simulink library "hal"  (Simulink 8.2)
settings: Solver=ode45  SolverMode=SingleTasking  StartTime=0.0  StopTime=10.0  RelTol=1e-3
PostLoadFcn:
  | , if any(exist('dsrtsu_mdlpostloadfcn', 'file') == [2, 3, 6]), try dsrtsu_mdlpostloadfcn('Execute', bdroot); catch fprintf('Error in PostLoadFcn (dsrtsu_mdlpostloadfcn) for model "%s":\n %s\n', bdroot, lasterr); end, end,
values from neighbouring files (symbols this model uses):
  INVALID_ABS1_TIMEOUT = single(0.03)    [hal_def.m]
  INVALID_ABS2_TIMEOUT = single(0.03)    [hal_def.m]
  INVALID_ABS3_TIMEOUT = single(0.03)    [hal_def.m]
  INVALID_ABS4_TIMEOUT = single(0.03)    [hal_def.m]
  INVALID_AC1_TIMEOUT = single(0.3)    [hal_def.m]
  INVALID_BCM1_TIMEOUT = single(0.6)    [hal_def.m]
  INVALID_BCM2_TIMEOUT = single(0.06)    [hal_def.m]
  INVALID_BOOSTER_VAC = uint32(255)    [hal_def.m]
  INVALID_CUR_VEHDECE = uint32(255)    [hal_def.m]
  INVALID_CURBRAKEDECE_REQ = uint32(255)    [hal_def.m]
  INVALID_CURSTEERANG_REQ = uint32(65535)    [hal_def.m]
  INVALID_CURSTEERTQ_REQ = uint32(255)    [hal_def.m]
  INVALID_ECM1_TIMEOUT = single(0.03)    [hal_def.m]
  INVALID_ECM2_TIMEOUT = single(0.03)    [hal_def.m]
  INVALID_ECM3_TIMEOUT = single(0.03)    [hal_def.m]
  INVALID_ECM9_TIMEOUT = single(0.03)    [hal_def.m]
  INVALID_ENG_TORQUE_FRICTIONAL = uint32(255)    [hal_def.m]
  INVALID_ENG_TORQUE_INDICATED = uint32(255)    [hal_def.m]
  INVALID_ENG_TORQUE_INDICATEDCOR = uint32(255)    [hal_def.m]
  INVALID_ENG_TQ_MAX = uint32(65535)    [hal_def.m]
  INVALID_ENG_TQ_MIN = uint32(65535)    [hal_def.m]
  INVALID_EPAS2_TIMEOUT = single(0.03)    [hal_def.m]
  INVALID_EPAS3_TIMEOUT = single(0.03)    [hal_def.m]
  INVALID_EPB1_TIMEOUT = single(0.12)    [hal_def.m]
  INVALID_EPS_BATTVOLT = uint32(251)    [hal_def.m]
  INVALID_ESC_BATTVOLT = uint32(251)    [hal_def.m]
  INVALID_GRADE = uint32(255)    [hal_def.m]
  INVALID_HCU3_TIMEOUT = single(0.03)    [hal_def.m]
  INVALID_HCU4_TIMEOUT = single(0.03)    [hal_def.m]
  INVALID_HMI1_TIMEOUT = single(0.03)    [hal_def.m]
  INVALID_HMI2_TIMEOUT = single(0.03)    [hal_def.m]
  INVALID_LAT_ACC = uint32(255)    [hal_def.m]
  INVALID_LONG_ACC = uint32(255)    [hal_def.m]
  INVALID_MC_PRESSURE = uint32(2047)    [hal_def.m]
  INVALID_METER1_TIMEOUT = single(0.3)    [hal_def.m]
  INVALID_METER3_TIMEOUT = single(0.3)    [hal_def.m]
  INVALID_METER_VEHSPD = uint32(2048)    [hal_def.m]
  INVALID_ODO_METER = uint32(1000000)    [hal_def.m]
  INVALID_OUTSIDE_TEMP = uint32(96)    [hal_def.m]
  INVALID_PARKBRAKEBIND_STAT = uint32(3)    [hal_def.m]
  INVALID_SAS1_TIMEOUT = single(0.03)    [hal_def.m]
  INVALID_SAS_ANGLE = uint32(65535)    [hal_def.m]
  INVALID_SHIFTER_POSN = uint32(6)    [hal_def.m]
  INVALID_TCM1_TIMEOUT = single(0.03)    [hal_def.m]
  INVALID_TCM2_TIMEOUT = single(0.03)    [hal_def.m]
  INVALID_VCU1_TIMEOUT = single(0.03)    [hal_def.m]
  INVALID_VCU2_TIMEOUT = single(0.03)    [hal_def.m]
  INVALID_VEH_CRASH = uint32(15)    [hal_def.m]
  INVALID_VEH_SPD = uint32(2048)    [hal_def.m]
  INVALID_WHEEL_SPD = uint32(16377)    [hal_def.m]
  INVALID_YAW_RATE = uint32(2001)    [hal_def.m]
undefined symbols (not defined in the file or in its folder): C_TASK_5MS_S, FALSE, INVALID_CURPTTORQ_REQ, KHAL_MssgIdObj1_num, KHAL_MssgIdObj2_num, KHAL_MssgIdObjStatus_num, TRUE
libraries: simulink x92
(part 6 of 8)

== system hal/dHAL_IN/dHAL_IN_ECM ==
  CAN1_Rx : Inport
  BO_790_ECM1_8_ECM : Subsystem
  BO_809_ECM2_8_ECM : Subsystem
  BO_821_ECM3_8_ECM : Subsystem
  BO_875_ECM9_8_ECM : Subsystem
  KFUN_AStpTimeMin_s1 : Constant  Value=INVALID_ENG_TORQUE_INDICATED
  KFUN_AStpTimeMin_s2 : Constant  Value=INVALID_ENG_TORQUE_INDICATEDCOR
  KFUN_AStpTimeMin_s3 : Constant  Value=INVALID_ENG_TORQUE_FRICTIONAL
  KFUN_AStpTimeMin_s5 : Constant  Value=INVALID_ENG_TQ_MAX
  KFUN_AStpTimeMin_s6 : Constant  Value=INVALID_ENG_TQ_MIN
  Relational Operator{1..3,5..6} (5 alike) : RelationalOperator  OutDataTypeStr=boolean
  VHAL_AccelPedalPosn_pct : Outport
  VHAL_AccelPedalPosnInvalid_flg : Outport  Port=2
  VHAL_EffAccelPedalPosn_pct : Outport  Port=3
  VHAL_EffAccelPedalPosnInvalid_flg : Outport  Port=4
  VHAL_CCEnable_flg : Outport  Port=5
  VHAL_CCEnableInvalid_flg : Outport  Port=6
  VHAL_CCActive_flg : Outport  Port=7
  VHAL_CCActiveInvalid_flg : Outport  Port=8
  VHAL_EngSpd_erpm : Outport  Port=9
  VHAL_EngSpdInvalid_flg : Outport  Port=10
  VHAL_EngTqIndicated_Nm : Outport  Port=11
  VHAL_EngTqIndicatedInvalid_flg : Outport  Port=12
  VHAL_EngTqIndicatedCOR_Nm : Outport  Port=13
  VHAL_EngTqIndicatedCORInvalid_flg : Outport  Port=14
  VHAL_EngTqUnCORFault_flg : Outport  Port=15
  VHAL_EngTqFriction_Nm : Outport  Port=16
  VHAL_EngTqFrictionInvalid_flg : Outport  Port=17
  VHAL_StandardTq_Nm : Outport  Port=18
  VHAL_EngTqMax_Nm : Outport  Port=19
  VHAL_EngTqMaxInvalid_flg : Outport  Port=20
  VHAL_EngTqMin_Nm : Outport  Port=21
  VHAL_EngTqMinInvalid_flg : Outport  Port=22
  VHAL_EMSHybridOpState_enum : Outport  Port=23
  VHAL_EMSOpState_enum : Outport  Port=24
  VHAL_ECM9RollCnt_cnt : Outport  Port=25
  VHAL_EngHoodOpen_flg : Outport  Port=26
  VHAL_EngRunning_flg : Outport  Port=27
  wires:
  BO_875_ECM9_8_ECM/7(EngTqMin_raw) -> Relational Operator6/1
  BO_875_ECM9_8_ECM/6(EngTqMin) -> VHAL_EngTqMin_Nm/1
  BO_875_ECM9_8_ECM/5(EngTqMax_raw) -> Relational Operator5/1
  BO_790_ECM1_8_ECM/7(CAN_TQI_ACOR_raw) -> Relational Operator2/1
  BO_790_ECM1_8_ECM/5(CAN_TQI_raw) -> Relational Operator1/1
  BO_790_ECM1_8_ECM/3(CAN_TQFR_raw) -> Relational Operator3/1
  KFUN_AStpTimeMin_s5/1 -> Relational Operator5/2
  KFUN_AStpTimeMin_s6/1 -> Relational Operator6/2
  KFUN_AStpTimeMin_s3/1 -> Relational Operator3/2
  KFUN_AStpTimeMin_s1/1 -> Relational Operator1/2
  KFUN_AStpTimeMin_s2/1 -> Relational Operator2/2
  BO_809_ECM2_8_ECM/1(Eng_Hood_SW) -> VHAL_EngHoodOpen_flg/1
  BO_809_ECM2_8_ECM/2(LV_CAN_ENG_RUN_ST) -> VHAL_EngRunning_flg/1
  [CAN1_Rx] -> BO_809_ECM2_8_ECM/1(CAN1_Rx)
  BO_875_ECM9_8_ECM/1(ECM9RollCnt) -> VHAL_ECM9RollCnt_cnt/1
  BO_875_ECM9_8_ECM/2(EMSHybridOpState) -> VHAL_EMSHybridOpState_enum/1
  BO_875_ECM9_8_ECM/3(EMSOpState) -> VHAL_EMSOpState_enum/1
  BO_875_ECM9_8_ECM/4(EngTqMax) -> VHAL_EngTqMax_Nm/1
  Relational Operator5/1 -> VHAL_EngTqMaxInvalid_flg/1
  Relational Operator6/1 -> VHAL_EngTqMinInvalid_flg/1
  [CAN1_Rx] -> BO_875_ECM9_8_ECM/1(CAN1_Rx1)
  Relational Operator3/1 -> VHAL_EngTqFrictionInvalid_flg/1
  BO_790_ECM1_8_ECM/2(CAN_TQFR) -> VHAL_EngTqFriction_Nm/1
  BO_790_ECM1_8_ECM/8(CAN_TQ_STND) -> VHAL_StandardTq_Nm/1
  BO_790_ECM1_8_ECM/9(LV_CAN_N_ERR) -> VHAL_EngSpdInvalid_flg/1
  BO_790_ECM1_8_ECM/1(CAN_N) -> VHAL_EngSpd_erpm/1
  Relational Operator1/1 -> VHAL_EngTqIndicatedInvalid_flg/1
  BO_790_ECM1_8_ECM/4(CAN_TQI) -> VHAL_EngTqIndicated_Nm/1
  BO_790_ECM1_8_ECM/6(CAN_TQI_ACOR) -> VHAL_EngTqIndicatedCOR_Nm/1
  Relational Operator2/1 -> VHAL_EngTqIndicatedCORInvalid_flg/1
  BO_790_ECM1_8_ECM/10(LV_CAN_SUB_TQI) -> VHAL_EngTqUnCORFault_flg/1
  [CAN1_Rx] -> BO_790_ECM1_8_ECM/1(CAN1_Rx)
  BO_821_ECM3_8_ECM/1(CAN_PV_AV) -> VHAL_AccelPedalPosn_pct/1
  BO_821_ECM3_8_ECM/2(CAN_PV_EFC) -> VHAL_EffAccelPedalPosn_pct/1
  BO_821_ECM3_8_ECM/3(LV_CAN_ERRPAS) -> VHAL_AccelPedalPosnInvalid_flg/1
  BO_821_ECM3_8_ECM/4(LV_CAN_ERRPVS) -> VHAL_EffAccelPedalPosnInvalid_flg/1
  BO_821_ECM3_8_ECM/5(LV_CAN_MAIN_CRU) -> VHAL_CCEnable_flg/1
  BO_821_ECM3_8_ECM/6(LV_CAN_MAIN_CRU_ER) -> VHAL_CCEnableInvalid_flg/1
  BO_821_ECM3_8_ECM/7(LV_CAN_SET_CRU) -> VHAL_CCActive_flg/1
  BO_821_ECM3_8_ECM/8(LV_CAN_SET_CRU_ERR) -> VHAL_CCActiveInvalid_flg/1
  [CAN1_Rx] -> BO_821_ECM3_8_ECM/1(CAN1_Rx)
  CAN1_Rx/1 -> [CAN1_Rx]

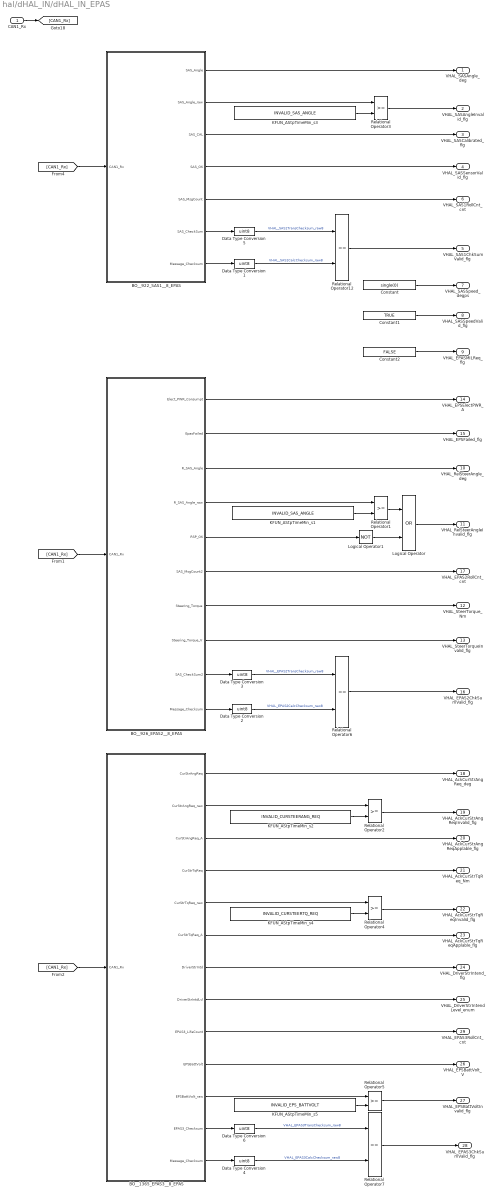
== system hal/dHAL_IN/dHAL_IN_EPAS ==
  CAN1_Rx : Inport
  BO__1365_EPAS3__8_EPAS : Subsystem
  BO__922_SAS1__8_EPAS : Subsystem
  BO__926_EPAS2__8_EPAS : Subsystem
  Constant : Constant  Value=single(0)
  Constant1 : Constant  Value=TRUE
  Constant2 : Constant  Value=FALSE
  Data Type Conversion{1..6} (6 alike) : DataTypeConversion  OutDataTypeStr=uint8
  KFUN_AStpTimeMin_s1 : Constant  Value=INVALID_SAS_ANGLE
  KFUN_AStpTimeMin_s2 : Constant  Value=INVALID_CURSTEERANG_REQ
  KFUN_AStpTimeMin_s3 : Constant  Value=INVALID_SAS_ANGLE
  KFUN_AStpTimeMin_s4 : Constant  Value=INVALID_CURSTEERTQ_REQ
  KFUN_AStpTimeMin_s5 : Constant  Value=INVALID_EPS_BATTVOLT
  Logical Operator : Logic  Operator=OR  AllPortsSameDT=off  OutDataTypeStr=boolean
  Logical Operator1 : Logic  Operator=NOT  AllPortsSameDT=off  OutDataTypeStr=boolean
  Relational Operator{1..5} (5 alike) : RelationalOperator  OutDataTypeStr=boolean
  Relational Operator12 : RelationalOperator  Operator===  OutDataTypeStr=boolean
  Relational Operator6 : RelationalOperator  Operator===  OutDataTypeStr=boolean
  Relational Operator7 : RelationalOperator  Operator===  OutDataTypeStr=boolean
  VHAL_SASAngle_deg : Outport
  VHAL_SASAngleInvalid_flg : Outport  Port=2
  VHAL_SASCalibrated_flg : Outport  Port=3
  VHAL_SASSensorValid_flg : Outport  Port=4
  VHAL_SAS1ChkSumValid_flg : Outport  Port=5
  VHAL_SAS1RollCnt_cnt : Outport  Port=6
  VHAL_SASSpeed_degps : Outport  Port=7
  VHAL_SASSpeedValid_flg : Outport  Port=8
  VHAL_EPASMILReq_flg : Outport  Port=9
  VHAL_RelSteerAngle_deg : Outport  Port=10
  VHAL_RelSteerAngleInvalid_flg : Outport  Port=11
  VHAL_SteerTorque_Nm : Outport  Port=12
  VHAL_SteerTorqueInvalid_flg : Outport  Port=13
  VHAL_EPSElectPWR_A : Outport  Port=14
  VHAL_EPSFailed_flg : Outport  Port=15
  VHAL_EPAS2ChkSumValid_flg : Outport  Port=16
  VHAL_EPAS2RollCnt_cnt : Outport  Port=17
  VHAL_AckCurStrAngReq_deg : Outport  Port=18
  VHAL_AckCurStrAngReqInvalid_flg : Outport  Port=19
  VHAL_AckCurStrAngReqApplable_flg : Outport  Port=20
  VHAL_AckCurStrTqReq_Nm : Outport  Port=21
  VHAL_AckCurStrTqReqInvalid_flg : Outport  Port=22
  VHAL_AckCurStrTqReqApplable_flg : Outport  Port=23
  VHAL_DriverStrIntend_flg : Outport  Port=24
  VHAL_DriverStrIntendLevel_enum : Outport  Port=25
  VHAL_EPSBattVolt_V : Outport  Port=26
  VHAL_EPSBattVoltInvalid_flg : Outport  Port=27
  VHAL_EPAS3ChkSumValid_flg : Outport  Port=28
  VHAL_EPAS3RollCnt_cnt : Outport  Port=29
  wires:
  BO__1365_EPAS3__8_EPAS/5(CurStrTqReq_raw) -> Relational Operator4/1
  BO__1365_EPAS3__8_EPAS/11(EPSBattVolt_raw) -> Relational Operator5/1
  BO__1365_EPAS3__8_EPAS/10(EPSBattVolt) -> VHAL_EPSBattVolt_V/1
  BO__1365_EPAS3__8_EPAS/2(CurStrAngReq_raw) -> Relational Operator2/1
  [CAN1_Rx] -> BO__1365_EPAS3__8_EPAS/1(CAN1_Rx)
  BO__926_EPAS2__8_EPAS/4(R_SAS_Angle_raw) -> Relational Operator1/1
  BO__922_SAS1__8_EPAS/2(SAS_Angle_raw) -> Relational Operator3/1
  [CAN1_Rx] -> BO__926_EPAS2__8_EPAS/1(CAN1_Rx)
  [CAN1_Rx] -> BO__922_SAS1__8_EPAS/1(CAN1_Rx)
  CAN1_Rx/1 -> [CAN1_Rx]
  BO__1365_EPAS3__8_EPAS/3(CurStrAngReq_A) -> VHAL_AckCurStrAngReqApplable_flg/1
  BO__1365_EPAS3__8_EPAS/13(Message_Checksum) -> Data Type Conversion4/1
  BO__1365_EPAS3__8_EPAS/12(EPAS3_Checksum) -> Data Type Conversion6/1
  Relational Operator7/1 -> VHAL_EPAS3ChkSumValid_flg/1
  Data Type Conversion4/1 -> Relational Operator7/2  "VHAL_EPAS3CalcChecksum_raw8"
  Data Type Conversion6/1 -> Relational Operator7/1  "VHAL_EPAS3TransChecksum_raw8"
  BO__926_EPAS2__8_EPAS/10(Message_Checksum) -> Data Type Conversion2/1
  BO__926_EPAS2__8_EPAS/9(SAS_CheckSum2) -> Data Type Conversion3/1
  Relational Operator6/1 -> VHAL_EPAS2ChkSumValid_flg/1
  Data Type Conversion2/1 -> Relational Operator6/2  "VHAL_EPAS2CalcChecksum_raw8"
  Data Type Conversion3/1 -> Relational Operator6/1  "VHAL_EPAS2TransChecksum_raw8"
  Relational Operator12/1 -> VHAL_SAS1ChkSumValid_flg/1
  Data Type Conversion1/1 -> Relational Operator12/2  "VHAL_SAS1CalcChecksum_raw8"
  Data Type Conversion5/1 -> Relational Operator12/1  "VHAL_SAS1TransChecksum_raw8"
  BO__922_SAS1__8_EPAS/7(Message_Checksum) -> Data Type Conversion1/1
  BO__922_SAS1__8_EPAS/6(SAS_CheckSum) -> Data Type Conversion5/1
  Relational Operator5/1 -> VHAL_EPSBattVoltInvalid_flg/1
  KFUN_AStpTimeMin_s5/1 -> Relational Operator5/2
  BO__1365_EPAS3__8_EPAS/8(DriverStrIntdLvl) -> VHAL_DriverStrIntendLevel_enum/1
  BO__1365_EPAS3__8_EPAS/7(DriverStrIntd) -> VHAL_DriverStrIntend_flg/1
  BO__1365_EPAS3__8_EPAS/4(CurStrTqReq) -> VHAL_AckCurStrTqReq_Nm/1
  BO__1365_EPAS3__8_EPAS/6(CurStrTqReq_A) -> VHAL_AckCurStrTqReqApplable_flg/1
  Relational Operator4/1 -> VHAL_AckCurStrTqReqInvalid_flg/1
  KFUN_AStpTimeMin_s4/1 -> Relational Operator4/2
  Relational Operator2/1 -> VHAL_AckCurStrAngReqInvalid_flg/1
  KFUN_AStpTimeMin_s2/1 -> Relational Operator2/2
  BO__1365_EPAS3__8_EPAS/1(CurStrAngReq) -> VHAL_AckCurStrAngReq_deg/1
  Logical Operator1/1 -> Logical Operator/2
  Logical Operator/1 -> VHAL_RelSteerAngleInvalid_flg/1
  Relational Operator1/1 -> Logical Operator/1
  KFUN_AStpTimeMin_s1/1 -> Relational Operator1/2
  BO__926_EPAS2__8_EPAS/3(R_SAS_Angle) -> VHAL_RelSteerAngle_deg/1
  Relational Operator3/1 -> VHAL_SASAngleInvalid_flg/1
  BO__922_SAS1__8_EPAS/1(SAS_Angle) -> VHAL_SASAngle_deg/1
  KFUN_AStpTimeMin_s3/1 -> Relational Operator3/2
  BO__926_EPAS2__8_EPAS/8(Steering_Torque_V) -> VHAL_SteerTorqueInvalid_flg/1
  BO__926_EPAS2__8_EPAS/7(Steering_Torque) -> VHAL_SteerTorque_Nm/1
  BO__926_EPAS2__8_EPAS/6(SAS_MsgCount2) -> VHAL_EPAS2RollCnt_cnt/1
  BO__926_EPAS2__8_EPAS/5(RSP_OK) -> Logical Operator1/1
  BO__926_EPAS2__8_EPAS/2(EpasFailed) -> VHAL_EPSFailed_flg/1
  BO__926_EPAS2__8_EPAS/1(Elect_PWR_Consumpt) -> VHAL_EPSElectPWR_A/1
  BO__1365_EPAS3__8_EPAS/9(EPAS3_LifeCount) -> VHAL_EPAS3RollCnt_cnt/1
  BO__922_SAS1__8_EPAS/4(SAS_OK) -> VHAL_SASSensorValid_flg/1
  BO__922_SAS1__8_EPAS/5(SAS_MsgCount) -> VHAL_SAS1RollCnt_cnt/1
  BO__922_SAS1__8_EPAS/3(SAS_CAL) -> VHAL_SASCalibrated_flg/1
  Constant/1 -> VHAL_SASSpeed_degps/1
  Constant1/1 -> VHAL_SASSpeedValid_flg/1
  Constant2/1 -> VHAL_EPASMILReq_flg/1

== system hal/dHAL_IN/dHAL_IN_HWIO ==
  IgnitionVolt_V : Constant  Value=12
  LFCEnableSw_flg : Constant  Value=0
  VbatprotVolt_V : Constant  Value=12
  VHAL_IgnitionVolt_V : Outport
  VHAL_VbatprotVolt_V : Outport  Port=2
  VHAL_LFCEnableSw_flg : Outport  Port=3
  wires:
  VbatprotVolt_V/1 -> VHAL_VbatprotVolt_V/1
  IgnitionVolt_V/1 -> VHAL_IgnitionVolt_V/1
  LFCEnableSw_flg/1 -> VHAL_LFCEnableSw_flg/1

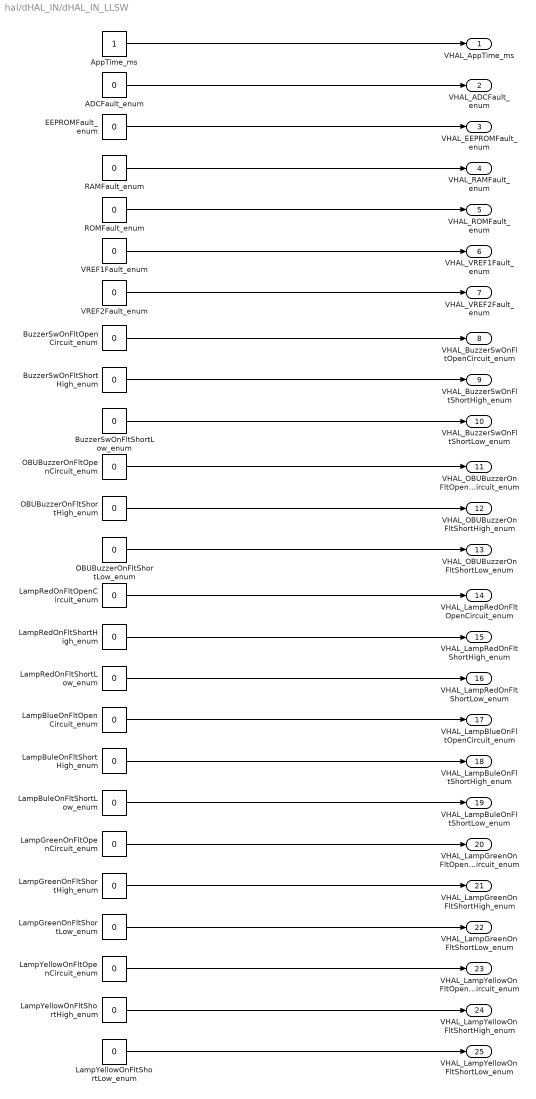
== system hal/dHAL_IN/dHAL_IN_LLSW ==
  ADCFault_enum : Constant  Value=0
  AppTime_ms : Constant
  BuzzerSwOnFltOpenCircuit_enum : Constant  Value=0
  BuzzerSwOnFltShortHigh_enum : Constant  Value=0
  BuzzerSwOnFltShortLow_enum : Constant  Value=0
  EEPROMFault_enum : Constant  Value=0
  LampBlueOnFltOpenCircuit_enum : Constant  Value=0
  LampBuleOnFltShortHigh_enum : Constant  Value=0
  LampBuleOnFltShortLow_enum : Constant  Value=0
  LampGreenOnFltOpenCircuit_enum : Constant  Value=0
  LampGreenOnFltShortHigh_enum : Constant  Value=0
  LampGreenOnFltShortLow_enum : Constant  Value=0
  LampRedOnFltOpenCircuit_enum : Constant  Value=0
  LampRedOnFltShortHigh_enum : Constant  Value=0
  LampRedOnFltShortLow_enum : Constant  Value=0
  LampYellowOnFltOpenCircuit_enum : Constant  Value=0
  LampYellowOnFltShortHigh_enum : Constant  Value=0
  LampYellowOnFltShortLow_enum : Constant  Value=0
  OBUBuzzerOnFltOpenCircuit_enum : Constant  Value=0
  OBUBuzzerOnFltShortHigh_enum : Constant  Value=0
  OBUBuzzerOnFltShortLow_enum : Constant  Value=0
  RAMFault_enum : Constant  Value=0
  ROMFault_enum : Constant  Value=0
  VREF1Fault_enum : Constant  Value=0
  VREF2Fault_enum : Constant  Value=0
  VHAL_AppTime_ms : Outport
  VHAL_ADCFault_enum : Outport  Port=2
  VHAL_EEPROMFault_enum : Outport  Port=3
  VHAL_RAMFault_enum : Outport  Port=4
  VHAL_ROMFault_enum : Outport  Port=5
  VHAL_VREF1Fault_enum : Outport  Port=6
  VHAL_VREF2Fault_enum : Outport  Port=7
  VHAL_BuzzerSwOnFltOpenCircuit_enum : Outport  Port=8
  VHAL_BuzzerSwOnFltShortHigh_enum : Outport  Port=9
  VHAL_BuzzerSwOnFltShortLow_enum : Outport  Port=10
  VHAL_OBUBuzzerOnFltOpenCircuit_enum : Outport  Port=11
  VHAL_OBUBuzzerOnFltShortHigh_enum : Outport  Port=12
  VHAL_OBUBuzzerOnFltShortLow_enum : Outport  Port=13
  VHAL_LampRedOnFltOpenCircuit_enum : Outport  Port=14
  VHAL_LampRedOnFltShortHigh_enum : Outport  Port=15
  VHAL_LampRedOnFltShortLow_enum : Outport  Port=16
  VHAL_LampBlueOnFltOpenCircuit_enum : Outport  Port=17
  VHAL_LampBuleOnFltShortHigh_enum : Outport  Port=18
  VHAL_LampBuleOnFltShortLow_enum : Outport  Port=19
  VHAL_LampGreenOnFltOpenCircuit_enum : Outport  Port=20
  VHAL_LampGreenOnFltShortHigh_enum : Outport  Port=21
  VHAL_LampGreenOnFltShortLow_enum : Outport  Port=22
  VHAL_LampYellowOnFltOpenCircuit_enum : Outport  Port=23
  VHAL_LampYellowOnFltShortHigh_enum : Outport  Port=24
  VHAL_LampYellowOnFltShortLow_enum : Outport  Port=25
  wires:
  LampYellowOnFltShortLow_enum/1 -> VHAL_LampYellowOnFltShortLow_enum/1
  LampYellowOnFltShortHigh_enum/1 -> VHAL_LampYellowOnFltShortHigh_enum/1
  LampYellowOnFltOpenCircuit_enum/1 -> VHAL_LampYellowOnFltOpenCircuit_enum/1
  LampGreenOnFltShortLow_enum/1 -> VHAL_LampGreenOnFltShortLow_enum/1
  LampGreenOnFltShortHigh_enum/1 -> VHAL_LampGreenOnFltShortHigh_enum/1
  LampGreenOnFltOpenCircuit_enum/1 -> VHAL_LampGreenOnFltOpenCircuit_enum/1
  LampBuleOnFltShortLow_enum/1 -> VHAL_LampBuleOnFltShortLow_enum/1
  LampBuleOnFltShortHigh_enum/1 -> VHAL_LampBuleOnFltShortHigh_enum/1
  LampBlueOnFltOpenCircuit_enum/1 -> VHAL_LampBlueOnFltOpenCircuit_enum/1
  LampRedOnFltShortLow_enum/1 -> VHAL_LampRedOnFltShortLow_enum/1
  LampRedOnFltShortHigh_enum/1 -> VHAL_LampRedOnFltShortHigh_enum/1
  LampRedOnFltOpenCircuit_enum/1 -> VHAL_LampRedOnFltOpenCircuit_enum/1
  OBUBuzzerOnFltShortLow_enum/1 -> VHAL_OBUBuzzerOnFltShortLow_enum/1
  OBUBuzzerOnFltShortHigh_enum/1 -> VHAL_OBUBuzzerOnFltShortHigh_enum/1
  OBUBuzzerOnFltOpenCircuit_enum/1 -> VHAL_OBUBuzzerOnFltOpenCircuit_enum/1
  BuzzerSwOnFltShortLow_enum/1 -> VHAL_BuzzerSwOnFltShortLow_enum/1
  BuzzerSwOnFltShortHigh_enum/1 -> VHAL_BuzzerSwOnFltShortHigh_enum/1
  BuzzerSwOnFltOpenCircuit_enum/1 -> VHAL_BuzzerSwOnFltOpenCircuit_enum/1
  ADCFault_enum/1 -> VHAL_ADCFault_enum/1
  AppTime_ms/1 -> VHAL_AppTime_ms/1
  EEPROMFault_enum/1 -> VHAL_EEPROMFault_enum/1
  RAMFault_enum/1 -> VHAL_RAMFault_enum/1
  ROMFault_enum/1 -> VHAL_ROMFault_enum/1
  VREF1Fault_enum/1 -> VHAL_VREF1Fault_enum/1
  VREF2Fault_enum/1 -> VHAL_VREF2Fault_enum/1

== system hal/dHAL_IN/dHAL_IN_METER ==
  CAN1_Rx : Inport
  BO__1104_Meter1__8_Meter : Subsystem
  BO__1306_Meter3__8_Meter : Subsystem
  KFUN_AStpTimeMin_s1 : Constant  Value=INVALID_METER_VEHSPD
  KFUN_AStpTimeMin_s5 : Constant  Value=INVALID_ODO_METER
  Relational Operator1 : RelationalOperator  OutDataTypeStr=boolean
  Relational Operator5 : RelationalOperator  OutDataTypeStr=boolean
  VHAL_OdoMeter_km : Outport
  VHAL_OdoMeterInvalid_flg : Outport  Port=2
  VHAL_LowBrakeFluid_flg : Outport  Port=3
  VHAL_ParkBrakeOn_flg : Outport  Port=4
  VHAL_SeatBeltNOTFasten_flg : Outport  Port=5
  VHAL_MeterVehSpd_kph : Outport  Port=6
  VHAL_MeterVehSpdInvalid_flg : Outport  Port=7
  wires:
  BO__1306_Meter3__8_Meter/2(Meter_Ind_VehSpeed_raw) -> Relational Operator1/1
  [CAN1_Rx] -> BO__1306_Meter3__8_Meter/1(CAN1_Rx)
  [CAN1_Rx] -> BO__1104_Meter1__8_Meter/1(CAN1_Rx)
  CAN1_Rx/1 -> [CAN1_Rx]
  BO__1104_Meter1__8_Meter/2(ODOMETER) -> VHAL_OdoMeter_km/1, Relational Operator5/1
  KFUN_AStpTimeMin_s5/1 -> Relational Operator5/2
  Relational Operator5/1 -> VHAL_OdoMeterInvalid_flg/1
  BO__1104_Meter1__8_Meter/1(LowBrakeFluid_Sta) -> VHAL_LowBrakeFluid_flg/1
  BO__1104_Meter1__8_Meter/3(ParkBrake) -> VHAL_ParkBrakeOn_flg/1
  BO__1104_Meter1__8_Meter/4(SeatBelt) -> VHAL_SeatBeltNOTFasten_flg/1
  KFUN_AStpTimeMin_s1/1 -> Relational Operator1/2
  BO__1306_Meter3__8_Meter/1(Meter_Ind_VehSpeed) -> VHAL_MeterVehSpd_kph/1
  Relational Operator1/1 -> VHAL_MeterVehSpdInvalid_flg/1

== system hal/dHAL_IN/dHAL_IN_TCM ==
  CAN1_Rx : Inport
  BO__832_TCM1__8_TCM : Subsystem
  BO__842_TCM2__8_TCM : Subsystem
  KFUN_AStpTimeMin_s3 : Constant  Value=INVALID_SHIFTER_POSN
  Relational Operator3 : RelationalOperator  Operator===  OutDataTypeStr=boolean
  VHAL_ShifterPosn_enum : Outport
  VHAL_ShifterPosnInvalid_flg : Outport  Port=2
  VHAL_NowGearPosn_enum : Outport  Port=3
  VHAL_NowGearPosnInvalid_flg : Outport  Port=4
  VHAL_TMTurbineSpd_rpm : Outport  Port=5
  VHAL_TMTurbineSpdInvalid_flg : Outport  Port=6
  VHAL_TCMFaultStatus_enum : Outport  Port=7
  VHAL_DriverMode_enum : Outport  Port=8
  wires:
  [CAN1_Rx] -> BO__842_TCM2__8_TCM/1(CAN1_Rx)
  [CAN1_Rx] -> BO__832_TCM1__8_TCM/1(CAN1_Rx)
  CAN1_Rx/1 -> [CAN1_Rx]
  BO__832_TCM1__8_TCM/2(CAN_GEAR_SEL_ETCU) -> VHAL_ShifterPosn_enum/1, Relational Operator3/1
  KFUN_AStpTimeMin_s3/1 -> Relational Operator3/2
  Relational Operator3/1 -> VHAL_ShifterPosnInvalid_flg/1
  BO__832_TCM1__8_TCM/3(CAN_GEAR_STATE_NOW) -> VHAL_NowGearPosn_enum/1
  BO__832_TCM1__8_TCM/4(CAN_GEAR_STA_NOW_V) -> VHAL_NowGearPosnInvalid_flg/1
  BO__832_TCM1__8_TCM/5(CAN_N_TM) -> VHAL_TMTurbineSpd_rpm/1
  BO__832_TCM1__8_TCM/6(LV_CAN_N_TM_ERR) -> VHAL_TMTurbineSpdInvalid_flg/1
  BO__832_TCM1__8_TCM/1(CAN_ETCU_STATE) -> VHAL_TCMFaultStatus_enum/1
  BO__842_TCM2__8_TCM/1(DR_MODE_IND) -> VHAL_DriverMode_enum/1

== system hal/dHAL_IN/HAL_IN_CANVALID/ChaekCANValid ==
  Rx_status : Inport
  TimeOut : Inport  Port=2
  Logical Operator : Logic  Operator=NOT  AllPortsSameDT=off  OutDataTypeStr=boolean
  Relational Operator : RelationalOperator  Operator=<=  OutDataTypeStr=boolean
  Timer : Subsystem  TreatAsAtomicUnit=on
  Valid_out : Outport
  wires:
  TimeOut/1 -> Relational Operator/2
  Relational Operator/1 -> Valid_out/1
  Logical Operator/1 -> Timer/Enable
  Rx_status/1 -> Logical Operator/1
  Timer/1(Timer (sec)) -> Relational Operator/1

== system hal/dHAL_IN/HAL_IN_CANVALID/ChaekCANValid1 ==
  Rx_status : Inport
  TimeOut : Inport  Port=2
  Logical Operator : Logic  Operator=NOT  AllPortsSameDT=off  OutDataTypeStr=boolean
  Relational Operator : RelationalOperator  Operator=<=  OutDataTypeStr=boolean
  Timer : Subsystem  TreatAsAtomicUnit=on
  Valid_out : Outport
  wires:
  Timer/1(Timer (sec)) -> Relational Operator/1
  Rx_status/1 -> Logical Operator/1
  Logical Operator/1 -> Timer/Enable
  Relational Operator/1 -> Valid_out/1
  TimeOut/1 -> Relational Operator/2

== system hal/dHAL_IN/HAL_IN_CANVALID/ChaekCANValid10 ==
  Rx_status : Inport
  TimeOut : Inport  Port=2
  Logical Operator : Logic  Operator=NOT  AllPortsSameDT=off  OutDataTypeStr=boolean
  Relational Operator : RelationalOperator  Operator=<=  OutDataTypeStr=boolean
  Timer : Subsystem  TreatAsAtomicUnit=on
  Valid_out : Outport
  wires:
  Timer/1(Timer (sec)) -> Relational Operator/1
  Rx_status/1 -> Logical Operator/1
  Logical Operator/1 -> Timer/Enable
  Relational Operator/1 -> Valid_out/1
  TimeOut/1 -> Relational Operator/2

== system hal/dHAL_IN/HAL_IN_CANVALID/ChaekCANValid11 ==
  Rx_status : Inport
  TimeOut : Inport  Port=2
  Logical Operator : Logic  Operator=NOT  AllPortsSameDT=off  OutDataTypeStr=boolean
  Relational Operator : RelationalOperator  Operator=<=  OutDataTypeStr=boolean
  Timer : Subsystem  TreatAsAtomicUnit=on
  Valid_out : Outport
  wires:
  TimeOut/1 -> Relational Operator/2
  Relational Operator/1 -> Valid_out/1
  Logical Operator/1 -> Timer/Enable
  Rx_status/1 -> Logical Operator/1
  Timer/1(Timer (sec)) -> Relational Operator/1

== system hal/dHAL_IN/HAL_IN_CANVALID/ChaekCANValid12 ==
  Rx_status : Inport
  TimeOut : Inport  Port=2
  Logical Operator : Logic  Operator=NOT  AllPortsSameDT=off  OutDataTypeStr=boolean
  Relational Operator : RelationalOperator  Operator=<=  OutDataTypeStr=boolean
  Timer : Subsystem  TreatAsAtomicUnit=on
  Valid_out : Outport
  wires:
  Timer/1(Timer (sec)) -> Relational Operator/1
  Rx_status/1 -> Logical Operator/1
  Logical Operator/1 -> Timer/Enable
  Relational Operator/1 -> Valid_out/1
  TimeOut/1 -> Relational Operator/2

== system hal/dHAL_IN/HAL_IN_CANVALID/ChaekCANValid13 ==
  Rx_status : Inport
  TimeOut : Inport  Port=2
  Logical Operator : Logic  Operator=NOT  AllPortsSameDT=off  OutDataTypeStr=boolean
  Relational Operator : RelationalOperator  Operator=<=  OutDataTypeStr=boolean
  Timer : Subsystem  TreatAsAtomicUnit=on
  Valid_out : Outport
  wires:
  TimeOut/1 -> Relational Operator/2
  Relational Operator/1 -> Valid_out/1
  Logical Operator/1 -> Timer/Enable
  Rx_status/1 -> Logical Operator/1
  Timer/1(Timer (sec)) -> Relational Operator/1

== system hal/dHAL_IN/HAL_IN_CANVALID/ChaekCANValid14 ==
  Rx_status : Inport
  TimeOut : Inport  Port=2
  Logical Operator : Logic  Operator=NOT  AllPortsSameDT=off  OutDataTypeStr=boolean
  Relational Operator : RelationalOperator  Operator=<=  OutDataTypeStr=boolean
  Timer : Subsystem  TreatAsAtomicUnit=on
  Valid_out : Outport
  wires:
  TimeOut/1 -> Relational Operator/2
  Relational Operator/1 -> Valid_out/1
  Logical Operator/1 -> Timer/Enable
  Rx_status/1 -> Logical Operator/1
  Timer/1(Timer (sec)) -> Relational Operator/1

== system hal/dHAL_IN/HAL_IN_CANVALID/ChaekCANValid15 ==
  Rx_status : Inport
  TimeOut : Inport  Port=2
  Logical Operator : Logic  Operator=NOT  AllPortsSameDT=off  OutDataTypeStr=boolean
  Relational Operator : RelationalOperator  Operator=<=  OutDataTypeStr=boolean
  Timer : Subsystem  TreatAsAtomicUnit=on
  Valid_out : Outport
  wires:
  Timer/1(Timer (sec)) -> Relational Operator/1
  Rx_status/1 -> Logical Operator/1
  Logical Operator/1 -> Timer/Enable
  Relational Operator/1 -> Valid_out/1
  TimeOut/1 -> Relational Operator/2

== system hal/dHAL_IN/HAL_IN_CANVALID/ChaekCANValid16 ==
  Rx_status : Inport
  TimeOut : Inport  Port=2
  Logical Operator : Logic  Operator=NOT  AllPortsSameDT=off  OutDataTypeStr=boolean
  Relational Operator : RelationalOperator  Operator=<=  OutDataTypeStr=boolean
  Timer : Subsystem  TreatAsAtomicUnit=on
  Valid_out : Outport
  wires:
  TimeOut/1 -> Relational Operator/2
  Relational Operator/1 -> Valid_out/1
  Logical Operator/1 -> Timer/Enable
  Rx_status/1 -> Logical Operator/1
  Timer/1(Timer (sec)) -> Relational Operator/1

== system hal/dHAL_IN/HAL_IN_CANVALID/ChaekCANValid17 ==
  Rx_status : Inport
  TimeOut : Inport  Port=2
  Logical Operator : Logic  Operator=NOT  AllPortsSameDT=off  OutDataTypeStr=boolean
  Relational Operator : RelationalOperator  Operator=<=  OutDataTypeStr=boolean
  Timer : Subsystem  TreatAsAtomicUnit=on
  Valid_out : Outport
  wires:
  TimeOut/1 -> Relational Operator/2
  Relational Operator/1 -> Valid_out/1
  Logical Operator/1 -> Timer/Enable
  Rx_status/1 -> Logical Operator/1
  Timer/1(Timer (sec)) -> Relational Operator/1

== system hal/dHAL_IN/HAL_IN_CANVALID/ChaekCANValid18 ==
  Rx_status : Inport
  TimeOut : Inport  Port=2
  Logical Operator : Logic  Operator=NOT  AllPortsSameDT=off  OutDataTypeStr=boolean
  Relational Operator : RelationalOperator  Operator=<=  OutDataTypeStr=boolean
  Timer : Subsystem  TreatAsAtomicUnit=on
  Valid_out : Outport
  wires:
  Timer/1(Timer (sec)) -> Relational Operator/1
  Rx_status/1 -> Logical Operator/1
  Logical Operator/1 -> Timer/Enable
  Relational Operator/1 -> Valid_out/1
  TimeOut/1 -> Relational Operator/2

== system hal/dHAL_IN/HAL_IN_CANVALID/ChaekCANValid19 ==
  Rx_status : Inport
  TimeOut : Inport  Port=2
  Logical Operator : Logic  Operator=NOT  AllPortsSameDT=off  OutDataTypeStr=boolean
  Relational Operator : RelationalOperator  Operator=<=  OutDataTypeStr=boolean
  Timer : Subsystem  TreatAsAtomicUnit=on
  Valid_out : Outport
  wires:
  TimeOut/1 -> Relational Operator/2
  Relational Operator/1 -> Valid_out/1
  Logical Operator/1 -> Timer/Enable
  Rx_status/1 -> Logical Operator/1
  Timer/1(Timer (sec)) -> Relational Operator/1

== system hal/dHAL_IN/HAL_IN_CANVALID/ChaekCANValid2 ==
  Rx_status : Inport
  TimeOut : Inport  Port=2
  Logical Operator : Logic  Operator=NOT  AllPortsSameDT=off  OutDataTypeStr=boolean
  Relational Operator : RelationalOperator  Operator=<=  OutDataTypeStr=boolean
  Timer : Subsystem  TreatAsAtomicUnit=on
  Valid_out : Outport
  wires:
  TimeOut/1 -> Relational Operator/2
  Relational Operator/1 -> Valid_out/1
  Logical Operator/1 -> Timer/Enable
  Rx_status/1 -> Logical Operator/1
  Timer/1(Timer (sec)) -> Relational Operator/1

== system hal/dHAL_IN/HAL_IN_CANVALID/ChaekCANValid20 ==
  Rx_status : Inport
  TimeOut : Inport  Port=2
  Logical Operator : Logic  Operator=NOT  AllPortsSameDT=off  OutDataTypeStr=boolean
  Relational Operator : RelationalOperator  Operator=<=  OutDataTypeStr=boolean
  Timer : Subsystem  TreatAsAtomicUnit=on
  Valid_out : Outport
  wires:
  Timer/1(Timer (sec)) -> Relational Operator/1
  Rx_status/1 -> Logical Operator/1
  Logical Operator/1 -> Timer/Enable
  Relational Operator/1 -> Valid_out/1
  TimeOut/1 -> Relational Operator/2

== system hal/dHAL_IN/HAL_IN_CANVALID/ChaekCANValid21 ==
  Rx_status : Inport
  TimeOut : Inport  Port=2
  Logical Operator : Logic  Operator=NOT  AllPortsSameDT=off  OutDataTypeStr=boolean
  Relational Operator : RelationalOperator  Operator=<=  OutDataTypeStr=boolean
  Timer : Subsystem  TreatAsAtomicUnit=on
  Valid_out : Outport
  wires:
  Timer/1(Timer (sec)) -> Relational Operator/1
  Rx_status/1 -> Logical Operator/1
  Logical Operator/1 -> Timer/Enable
  Relational Operator/1 -> Valid_out/1
  TimeOut/1 -> Relational Operator/2

== system hal/dHAL_IN/HAL_IN_CANVALID/ChaekCANValid22 ==
  Rx_status : Inport
  TimeOut : Inport  Port=2
  Logical Operator : Logic  Operator=NOT  AllPortsSameDT=off  OutDataTypeStr=boolean
  Relational Operator : RelationalOperator  Operator=<=  OutDataTypeStr=boolean
  Timer : Subsystem  TreatAsAtomicUnit=on
  Valid_out : Outport
  wires:
  TimeOut/1 -> Relational Operator/2
  Relational Operator/1 -> Valid_out/1
  Logical Operator/1 -> Timer/Enable
  Rx_status/1 -> Logical Operator/1
  Timer/1(Timer (sec)) -> Relational Operator/1

== system hal/dHAL_IN/HAL_IN_CANVALID/ChaekCANValid23 ==
  Rx_status : Inport
  TimeOut : Inport  Port=2
  Logical Operator : Logic  Operator=NOT  AllPortsSameDT=off  OutDataTypeStr=boolean
  Relational Operator : RelationalOperator  Operator=<=  OutDataTypeStr=boolean
  Timer : Subsystem  TreatAsAtomicUnit=on
  Valid_out : Outport
  wires:
  Timer/1(Timer (sec)) -> Relational Operator/1
  Rx_status/1 -> Logical Operator/1
  Logical Operator/1 -> Timer/Enable
  Relational Operator/1 -> Valid_out/1
  TimeOut/1 -> Relational Operator/2

== system hal/dHAL_IN/HAL_IN_CANVALID/ChaekCANValid24 ==
  Rx_status : Inport
  TimeOut : Inport  Port=2
  Logical Operator : Logic  Operator=NOT  AllPortsSameDT=off  OutDataTypeStr=boolean
  Relational Operator : RelationalOperator  Operator=<=  OutDataTypeStr=boolean
  Timer : Subsystem  TreatAsAtomicUnit=on
  Valid_out : Outport
  wires:
  Timer/1(Timer (sec)) -> Relational Operator/1
  Rx_status/1 -> Logical Operator/1
  Logical Operator/1 -> Timer/Enable
  Relational Operator/1 -> Valid_out/1
  TimeOut/1 -> Relational Operator/2

== system hal/dHAL_IN/HAL_IN_CANVALID/ChaekCANValid3 ==
  Rx_status : Inport
  TimeOut : Inport  Port=2
  Logical Operator : Logic  Operator=NOT  AllPortsSameDT=off  OutDataTypeStr=boolean
  Relational Operator : RelationalOperator  Operator=<=  OutDataTypeStr=boolean
  Timer : Subsystem  TreatAsAtomicUnit=on
  Valid_out : Outport
  wires:
  Timer/1(Timer (sec)) -> Relational Operator/1
  Rx_status/1 -> Logical Operator/1
  Logical Operator/1 -> Timer/Enable
  Relational Operator/1 -> Valid_out/1
  TimeOut/1 -> Relational Operator/2

== system hal/dHAL_IN/HAL_IN_CANVALID/ChaekCANValid4 ==
  Rx_status : Inport
  TimeOut : Inport  Port=2
  Logical Operator : Logic  Operator=NOT  AllPortsSameDT=off  OutDataTypeStr=boolean
  Relational Operator : RelationalOperator  Operator=<=  OutDataTypeStr=boolean
  Timer : Subsystem  TreatAsAtomicUnit=on
  Valid_out : Outport
  wires:
  TimeOut/1 -> Relational Operator/2
  Relational Operator/1 -> Valid_out/1
  Logical Operator/1 -> Timer/Enable
  Rx_status/1 -> Logical Operator/1
  Timer/1(Timer (sec)) -> Relational Operator/1

== system hal/dHAL_IN/HAL_IN_CANVALID/ChaekCANValid5 ==
  Rx_status : Inport
  TimeOut : Inport  Port=2
  Logical Operator : Logic  Operator=NOT  AllPortsSameDT=off  OutDataTypeStr=boolean
  Relational Operator : RelationalOperator  Operator=<=  OutDataTypeStr=boolean
  Timer : Subsystem  TreatAsAtomicUnit=on
  Valid_out : Outport
  wires:
  Timer/1(Timer (sec)) -> Relational Operator/1
  Rx_status/1 -> Logical Operator/1
  Logical Operator/1 -> Timer/Enable
  Relational Operator/1 -> Valid_out/1
  TimeOut/1 -> Relational Operator/2

== system hal/dHAL_IN/HAL_IN_CANVALID/ChaekCANValid6 ==
  Rx_status : Inport
  TimeOut : Inport  Port=2
  Logical Operator : Logic  Operator=NOT  AllPortsSameDT=off  OutDataTypeStr=boolean
  Relational Operator : RelationalOperator  Operator=<=  OutDataTypeStr=boolean
  Timer : Subsystem  TreatAsAtomicUnit=on
  Valid_out : Outport
  wires:
  TimeOut/1 -> Relational Operator/2
  Relational Operator/1 -> Valid_out/1
  Logical Operator/1 -> Timer/Enable
  Rx_status/1 -> Logical Operator/1
  Timer/1(Timer (sec)) -> Relational Operator/1

== system hal/dHAL_IN/HAL_IN_CANVALID/ChaekCANValid7 ==
  Rx_status : Inport
  TimeOut : Inport  Port=2
  Logical Operator : Logic  Operator=NOT  AllPortsSameDT=off  OutDataTypeStr=boolean
  Relational Operator : RelationalOperator  Operator=<=  OutDataTypeStr=boolean
  Timer : Subsystem  TreatAsAtomicUnit=on
  Valid_out : Outport
  wires:
  Timer/1(Timer (sec)) -> Relational Operator/1
  Rx_status/1 -> Logical Operator/1
  Logical Operator/1 -> Timer/Enable
  Relational Operator/1 -> Valid_out/1
  TimeOut/1 -> Relational Operator/2

== system hal/dHAL_IN/HAL_IN_CANVALID/ChaekCANValid8 ==
  Rx_status : Inport
  TimeOut : Inport  Port=2
  Logical Operator : Logic  Operator=NOT  AllPortsSameDT=off  OutDataTypeStr=boolean
  Relational Operator : RelationalOperator  Operator=<=  OutDataTypeStr=boolean
  Timer : Subsystem  TreatAsAtomicUnit=on
  Valid_out : Outport
  wires:
  Timer/1(Timer (sec)) -> Relational Operator/1
  Rx_status/1 -> Logical Operator/1
  Logical Operator/1 -> Timer/Enable
  Relational Operator/1 -> Valid_out/1
  TimeOut/1 -> Relational Operator/2

== system hal/dHAL_IN/HAL_IN_CANVALID/ChaekCANValid9 ==
  Rx_status : Inport
  TimeOut : Inport  Port=2
  Logical Operator : Logic  Operator=NOT  AllPortsSameDT=off  OutDataTypeStr=boolean
  Relational Operator : RelationalOperator  Operator=<=  OutDataTypeStr=boolean
  Timer : Subsystem  TreatAsAtomicUnit=on
  Valid_out : Outport
  wires:
  TimeOut/1 -> Relational Operator/2
  Relational Operator/1 -> Valid_out/1
  Logical Operator/1 -> Timer/Enable
  Rx_status/1 -> Logical Operator/1
  Timer/1(Timer (sec)) -> Relational Operator/1

== system hal/dHAL_IN/HAL_IN_EPB/BO__928_EPB1__8_EPB ==
  CAN1_Rx : Inport
  Bus Selector : BusSelector  OutputSignals=EPB1.PB_BrakeBinStat
  PB_BrakeBinStat : Outport
  wires:
  Bus Selector/1 -> PB_BrakeBinStat/1  "<PB_BrakeBinStat>"
  CAN1_Rx/1 -> [CAN1_Rx]
  [CAN1_Rx] -> Bus Selector/1

== system hal/dHAL_IN/HAL_IN_HMI/BO__1347_HMI1__8_HMI ==
  CAN1_Rx : Inport
  Bus Selector : BusSelector  OutputSignals=HMI1.ACCCancel,HMI1.ACCOn,HMI1.ACCRes_SpdInc,HMI1.ACCSet_SpdDec,HMI1.ACCSpeedDec,HMI1.ACCSpeedInc,HMI1.ACCTimeGapDec,HMI1.ACCTimeGapInc,HMI1.AEBEnable,HMI1.CSCEnable,HMI1.FCWEnable,HMI1.IGSAOn,HMI1.IGSARes_SpdInc,HMI1.IGSASet_SpdDec,HMI1.IGSASwitchMode,HMI1.LCSEnable,HMI1.LFC_PilotCancel,HMI1.LFC_PilotOn,HMI1.LKAEnable,HMI1.MAPAEnable,HMI1.FCWWarningMode,HMI1.DefMaxACCSetSpeed
  ACCCancel : Outport
  ACCOn : Outport  Port=2
  ACCRes_SpdInc : Outport  Port=3
  ACCSet_SpdDec : Outport  Port=4
  ACCSpeedDec : Outport  Port=5
  ACCSpeedInc : Outport  Port=6
  ACCTimeGapDec : Outport  Port=7
  ACCTimeGapInc : Outport  Port=8
  AEBEnable : Outport  Port=9
  CSCEnable : Outport  Port=10
  FCWEnable : Outport  Port=11
  IGSAOn : Outport  Port=12
  IGSARes_SpdInc : Outport  Port=13
  IGSASet_SpdDec : Outport  Port=14
  IGSASwitchMode : Outport  Port=15
  LCSEnable : Outport  Port=16
  LFC_PilotCancel : Outport  Port=17
  LFC_PilotOn : Outport  Port=18
  LKAEnable : Outport  Port=19
  MAPAEnable : Outport  Port=20
  FCWWarningMode : Outport  Port=21
  DefMaxACCSetSpeed : Outport  Port=22
  wires:
  Bus Selector/22 -> DefMaxACCSetSpeed/1  "<DefMaxACCSetSpeed>"
  Bus Selector/21 -> FCWWarningMode/1  "<FCWWarningMode>"
  Bus Selector/15 -> IGSASwitchMode/1  "<IGSASwitchMode>"
  Bus Selector/14 -> IGSASet_SpdDec/1  "<IGSASet_SpdDec>"
  Bus Selector/13 -> IGSARes_SpdInc/1  "<IGSARes_SpdInc>"
  Bus Selector/12 -> IGSAOn/1  "<IGSAOn>"
  Bus Selector/20 -> MAPAEnable/1  "<MAPAEnable>"
  Bus Selector/19 -> LKAEnable/1  "<LKAEnable>"
  Bus Selector/18 -> LFC_PilotOn/1  "<LFC_PilotOn>"
  Bus Selector/17 -> LFC_PilotCancel/1  "<LFC_PilotCancel>"
  Bus Selector/16 -> LCSEnable/1  "<LCSEnable>"
  Bus Selector/11 -> FCWEnable/1  "<FCWEnable>"
  Bus Selector/10 -> CSCEnable/1  "<CSCEnable>"
  Bus Selector/9 -> AEBEnable/1  "<AEBEnable>"
  Bus Selector/8 -> ACCTimeGapInc/1  "<ACCTimeGapInc>"
  Bus Selector/7 -> ACCTimeGapDec/1  "<ACCTimeGapDec>"
  Bus Selector/6 -> ACCSpeedInc/1  "<ACCSpeedInc>"
  Bus Selector/5 -> ACCSpeedDec/1  "<ACCSpeedDec>"
  Bus Selector/4 -> ACCSet_SpdDec/1  "<ACCSet_SpdDec>"
  Bus Selector/3 -> ACCRes_SpdInc/1  "<ACCRes_SpdInc>"
  Bus Selector/2 -> ACCOn/1  "<ACCOn>"
  Bus Selector/1 -> ACCCancel/1  "<ACCCancel>"
  CAN1_Rx/1 -> [CAN1_Rx]
  [CAN1_Rx] -> Bus Selector/1

== system hal/dHAL_IN/HAL_IN_RadObjDecoder/RObj_Parser ==
  RObj_Status : Inport
  RObj_Frames1 : Inport  Port=2
  RObj_Frames2 : Inport  Port=3
  RObj_CollDetWarn : Inport  Port=4
  Ground : Ground
  Ground1 : Ground
  RObj_FramesParser : MATLAB Function  TreatAsAtomicUnit=on
  RObj_StatusParser : MATLAB Function  TreatAsAtomicUnit=on
  Terminator : Terminator
  VHAL_RadNofObjects_num : Outport
  VHAL_MeasCounter_num : Outport  Port=2
  VHAL_SensorRxInvalid_enum : Outport  Port=3
  VHAL_SensorSupplyVoltage_V : Outport  Port=4
  VHAL_SensorDefective_enum : Outport  Port=5
  VHAL_SensorMisaligned_enum : Outport  Port=6
  VHAL_SensorSwitchedOff_enum : Outport  Port=7
  VHAL_SensorExternalDisturbed_enum : Outport  Port=8
  VHAL_SensorOutputReduced_enum : Outport  Port=9
  VHAL_LatDistToborderLeft_m : Outport  Port=10
  VHAL_LatDistToborderRight_m : Outport  Port=11
  VHAL_RadObjRolCountVect40_num : Outport  Port=12
  VHAL_RadObjIDVect40_num : Outport  Port=13
  VHAL_RadObjXDisplVect40_m : Outport  Port=14
  VHAL_RadObjVrelXVect40_mps : Outport  Port=15
  VHAL_RadObjAccelXVect40_mps2 : Outport  Port=16
  VHAL_RadObjYDisplVect40_m : Outport  Port=17
  VHAL_RadObjDynPropVect40_enum : Outport  Port=18
  VHAL_RadObjPExistVect40_enum : Outport  Port=19
  VHAL_RadObjMeasStatVect40_enum : Outport  Port=20
  VHAL_RadObjWidthVect40_m : Outport  Port=21
  VHAL_RadObjLengthVect40_m : Outport  Port=22
  VHAL_RadObjRCSVect40_num : Outport  Port=23
  VHAL_RadObjVrelYVect40_mps : Outport  Port=24
  VHAL_RadObjProbVect40_num : Outport  Port=25
  VHAL_RadWarningLevel_enum : Outport  Port=26
  VHAL_RadWarningObjID_num : Outport  Port=27
  wires:
  Ground1/1 -> VHAL_RadWarningObjID_num/1
  Ground/1 -> VHAL_RadWarningLevel_enum/1
  RObj_CollDetWarn/1 -> Terminator/1
  RObj_StatusParser/4(SensorSupplyVoltage) -> VHAL_SensorSupplyVoltage_V/1
  RObj_StatusParser/3(SensorRxInvalid) -> VHAL_SensorRxInvalid_enum/1
  RObj_StatusParser/10(LatDistToborderLeft) -> VHAL_LatDistToborderLeft_m/1
  RObj_StatusParser/2(MeasCounter) -> VHAL_MeasCounter_num/1
  RObj_StatusParser/11(LatDistToborderRight) -> VHAL_LatDistToborderRight_m/1
  RObj_StatusParser/9(SensorOutputReduced) -> VHAL_SensorOutputReduced_enum/1
  RObj_StatusParser/7(SensorSwitchedOff) -> VHAL_SensorSwitchedOff_enum/1
  RObj_StatusParser/8(SensorExternalDisturbed) -> VHAL_SensorExternalDisturbed_enum/1
  RObj_StatusParser/5(SensorDefective) -> VHAL_SensorDefective_enum/1
  RObj_StatusParser/6(SensorMisaligned) -> VHAL_SensorMisaligned_enum/1
  RObj_StatusParser/1(N_of_Objects) -> VHAL_RadNofObjects_num/1
  RObj_Frames2/1 -> RObj_FramesParser/2(Frames2)
  RObj_Frames1/1 -> RObj_FramesParser/1(Frames1)
  RObj_FramesParser/13(Obj_LatSpeed) -> VHAL_RadObjVrelYVect40_mps/1
  RObj_FramesParser/12(Obj_RCSValue) -> VHAL_RadObjRCSVect40_num/1
  RObj_FramesParser/14(Obj_ObstacleProb) -> VHAL_RadObjProbVect40_num/1
  RObj_FramesParser/10(Obj_Width) -> VHAL_RadObjWidthVect40_m/1
  RObj_FramesParser/8(Obj_ProbOfExist) -> VHAL_RadObjPExistVect40_enum/1
  RObj_FramesParser/11(Obj_Length) -> VHAL_RadObjLengthVect40_m/1
  RObj_FramesParser/9(Obj_MeasStat) -> VHAL_RadObjMeasStatVect40_enum/1
  RObj_FramesParser/7(Obj_DynProp) -> VHAL_RadObjDynPropVect40_enum/1
  RObj_FramesParser/6(Obj_LatDispl) -> VHAL_RadObjYDisplVect40_m/1
  RObj_FramesParser/5(Obj_AccelLong) -> VHAL_RadObjAccelXVect40_mps2/1
  RObj_FramesParser/4(Obj_VrelLong) -> VHAL_RadObjVrelXVect40_mps/1
  RObj_FramesParser/3(Obj_LongDispl) -> VHAL_RadObjXDisplVect40_m/1
  RObj_FramesParser/2(Obj_ID) -> VHAL_RadObjIDVect40_num/1
  RObj_FramesParser/1(Obj_RolCount) -> VHAL_RadObjRolCountVect40_num/1
  RObj_Status/1 -> RObj_StatusParser/1(Status_Frame)

== system hal/dHAL_IN/HAL_IN_RadObjDecoder/RObjectPackFrame ==
  CAN_Frames : Inport
  CaptureMessage1 : Inport  Port=2
  CaptureMessage2 : Inport  Port=3
  CaptureMessage3 : Inport  Port=4
  CaptureMessage4 : Inport  Port=5
  CaptureMessage5 : Inport  Port=6
  CaptureMessage6 : Inport  Port=7
  CaptureMessage7 : Inport  Port=8
  CaptureMessage8 : Inport  Port=9
  CaptureMessage9 : Inport  Port=10
  CaptureMessage10 : Inport  Port=11
  CaptureMessage11 : Inport  Port=12
  CaptureMessage12 : Inport  Port=13
  CaptureMessage13 : Inport  Port=14
  CaptureMessage14 : Inport  Port=15
  CaptureMessage15 : Inport  Port=16
  CaptureMessage16 : Inport  Port=17
  CaptureMessage17 : Inport  Port=18
  CaptureMessage18 : Inport  Port=19
  CaptureMessage19 : Inport  Port=20
  CaptureMessage20 : Inport  Port=21
  CaptureMessage21 : Inport  Port=22
  CaptureMessage22 : Inport  Port=23
  CaptureMessage23 : Inport  Port=24
  CaptureMessage24 : Inport  Port=25
  CaptureMessage25 : Inport  Port=26
  Bus Selector5 : BusSelector  OutputSignals=Status,ID,RAW_Byte_1,RAW_Byte_2,RAW_Byte_3,RAW_Byte_4,RAW_Byte_5,RAW_Byte_6,RAW_Byte_7,RAW_Byte_8
  Delay : Delay  DelayLength=1  InitialCondition=0
  For Iterator : ForIterator  IterationSource=external  IterationLimit=25
  Multiport Switch : MultiPortSwitch  Inputs=25
  RObjects_Decoder_v2 : Subsystem
  R_Objects_out : Outport  OutDataTypeStr=Bus: R_Objects
  wires:
  CAN_Frames/1 -> For Iterator/1
  Delay/1 -> RObjects_Decoder_v2/11(R_Objects_in)
  Bus Selector5/6 -> RObjects_Decoder_v2/6(Byte4)  "<RAW_Byte_4>"
  Bus Selector5/7 -> RObjects_Decoder_v2/7(Byte5)  "<RAW_Byte_5>"
  Bus Selector5/5 -> RObjects_Decoder_v2/5(Byte3)  "<RAW_Byte_3>"
  Bus Selector5/9 -> RObjects_Decoder_v2/9(Byte7)  "<RAW_Byte_7>"
  Bus Selector5/8 -> RObjects_Decoder_v2/8(Byte6)  "<RAW_Byte_6>"
  Bus Selector5/1 -> RObjects_Decoder_v2/1(Status)  "<Status>"
  Bus Selector5/10 -> RObjects_Decoder_v2/10(Byte8)  "<RAW_Byte_8>"
  Bus Selector5/3 -> RObjects_Decoder_v2/3(Byte1)  "<RAW_Byte_1>"
  Bus Selector5/4 -> RObjects_Decoder_v2/4(Byte2)  "<RAW_Byte_2>"
  Bus Selector5/2 -> RObjects_Decoder_v2/2(ID)  "<ID>"
  Multiport Switch/1 -> Bus Selector5/1
  RObjects_Decoder_v2/1(R_Objects_out) -> R_Objects_out/1, Delay/1
  CaptureMessage25/1 -> Multiport Switch/26
  CaptureMessage24/1 -> Multiport Switch/25
  CaptureMessage23/1 -> Multiport Switch/24
  CaptureMessage22/1 -> Multiport Switch/23
  CaptureMessage21/1 -> Multiport Switch/22
  CaptureMessage20/1 -> Multiport Switch/21
  CaptureMessage19/1 -> Multiport Switch/20
  CaptureMessage18/1 -> Multiport Switch/19
  CaptureMessage17/1 -> Multiport Switch/18
  CaptureMessage16/1 -> Multiport Switch/17
  CaptureMessage15/1 -> Multiport Switch/16
  CaptureMessage14/1 -> Multiport Switch/15
  CaptureMessage13/1 -> Multiport Switch/14
  CaptureMessage12/1 -> Multiport Switch/13
  CaptureMessage11/1 -> Multiport Switch/12
  CaptureMessage10/1 -> Multiport Switch/11
  CaptureMessage9/1 -> Multiport Switch/10
  CaptureMessage8/1 -> Multiport Switch/9
  CaptureMessage7/1 -> Multiport Switch/8
  CaptureMessage6/1 -> Multiport Switch/7
  CaptureMessage5/1 -> Multiport Switch/6
  CaptureMessage4/1 -> Multiport Switch/5
  CaptureMessage3/1 -> Multiport Switch/4
  CaptureMessage2/1 -> Multiport Switch/3
  For Iterator/1 -> Multiport Switch/1
  CaptureMessage1/1 -> Multiport Switch/2

== system hal/dHAL_IN/HAL_IN_VCU/BO__1344_HMI2__8_VCU ==
  CAN1_Rx : Inport
  Bus Selector : BusSelector  OutputSignals=HMI2.ACCOn_VCU,HMI2.ACCRes_SpdInc_VCU,HMI2.ACCSet_SpdDec_VCU,HMI2.ACCTimeGapInc_VCU,HMI2.ACCTimeGapDec_VCU,HMI2.LFCOn_VCU,HMI2.MSAOn_VCU
  ACCOn_VCU : Outport
  ACCRes_SpdInc_VCU : Outport  Port=2
  ACCSet_SpdDec_VCU : Outport  Port=3
  ACCTimeGapInc_VCU : Outport  Port=4
  ACCTimeGapDec_VCU : Outport  Port=5
  LFCOn_VCU : Outport  Port=6
  MSAOn_VCU : Outport  Port=7
  wires:
  Bus Selector/7 -> MSAOn_VCU/1  "<MSAOn_VCU>"
  Bus Selector/6 -> LFCOn_VCU/1  "<LFCOn_VCU>"
  Bus Selector/5 -> ACCTimeGapDec_VCU/1  "<ACCTimeGapDec_VCU>"
  Bus Selector/4 -> ACCTimeGapInc_VCU/1  "<ACCTimeGapInc_VCU>"
  Bus Selector/3 -> ACCSet_SpdDec_VCU/1  "<ACCSet_SpdDec_VCU>"
  Bus Selector/2 -> ACCRes_SpdInc_VCU/1  "<ACCRes_SpdInc_VCU>"
  Bus Selector/1 -> ACCOn_VCU/1  "<ACCOn_VCU>"
  [CAN1_Rx] -> Bus Selector/1
  CAN1_Rx/1 -> [CAN1_Rx]

== system hal/dHAL_IN/HAL_IN_VCU/BO__1360_VCU1__8_VCU ==
  CAN1_Rx : Inport
  Bitwise Operator : simulink/Logic and Bit Operations/Bitwise Operator  logicop=AND  UseBitMask=on  BitMask=bin2dec('11110000')  BitMaskRealWorld=Stored Integer
  Bus Selector : BusSelector  OutputSignals=VCU1.BrakePrefillAvail,VCU1.CurBrakDecReq,VCU1.CurBrakDecReq_A,VCU1.CurEngTqReq,VCU1.CurEngTqReq_A,VCU1.CurVehDec,VCU1.CurVehDec_V,VCU1.DecContMan,VCU1.DrivBrakSw,VCU1.EMSExtTqAvail,VCU1.EMSTqSrc,VCU1.ESCBrakStatus,VCU1.ESCExtBrkAvail,VCU1.VCUFault,VCU1.VCUBattVolt,VCU1.VCU1_Checksum,VCU1.VCU1_LifeCount
  Bus Selector1 : BusSelector  OutputSignals=VCU1.RAW_Byte_5,VCU1.RAW_Byte_2,VCU1.RAW_Byte_1,VCU1.RAW_Byte_6,VCU1.RAW_Byte_7
  ChecksumCalculation : Subsystem  TreatAsAtomicUnit=on
  IcM : Subsystem  TreatAsAtomicUnit=on
  BrakePrefillAvail : Outport
  CurBrakDecReq : Outport  Port=2
  CurBrakDecReq_raw : Outport  Port=3
  CurBrakDecReq_A : Outport  Port=4
  CurEngTqReq : Outport  Port=5
  CurEngTqReq_raw : Outport  Port=6
  CurEngTqReq_A : Outport  Port=7
  CurVehDec : Outport  Port=8
  CurVehDec_raw : Outport  Port=9
  CurVehDec_V : Outport  Port=10
  DecContMan : Outport  Port=11
  DrivBrakSw : Outport  Port=12
  EMSExtTqAvail : Outport  Port=13
  EMSTqSrc : Outport  Port=14
  ESCBrakStatus : Outport  Port=15
  ESCExtBrkAvail : Outport  Port=16
  VCUFault : Outport  Port=17
  VCUBattVolt : Outport  Port=18
  VCUBattVolt_raw : Outport  Port=19
  VCU1_LifeCount : Outport  Port=20
  VCU1_Checksum : Outport  Port=21
  Message_Checksum : Outport  Port=22
  wires:
  ChecksumCalculation/1(Message_Checksum) -> Message_Checksum/1
  [CAN1_Rx] -> ChecksumCalculation/1(CAN1_Rx)
  Bus Selector1/5 -> VCUBattVolt_raw/1  "<RAW_Byte_7>"
  Bus Selector1/4 -> CurVehDec_raw/1  "<RAW_Byte_6>"
  Bus Selector1/1 -> CurBrakDecReq_raw/1  "<RAW_Byte_5>"
  Bus Selector1/3 -> IcM/2(HighByte)  "<RAW_Byte_1>"
  Bus Selector1/2 -> Bitwise Operator/1  "<RAW_Byte_2>"
  IcM/1(HighLowByte) -> CurEngTqReq_raw/1
  Bitwise Operator/1 -> IcM/1(LowByte)
  [CAN1_Rx] -> Bus Selector1/1
  Bus Selector/5 -> CurEngTqReq_A/1  "<CurEngTqReq_A>"
  Bus Selector/3 -> CurBrakDecReq_A/1  "<CurBrakDecReq_A>"
  Bus Selector/15 -> VCUBattVolt/1  "<VCUBattVolt>"
  Bus Selector/17 -> VCU1_LifeCount/1  "<VCU1_LifeCount>"
  Bus Selector/16 -> VCU1_Checksum/1  "<VCU1_Checksum>"
  Bus Selector/14 -> VCUFault/1  "<VCUFault>"
  Bus Selector/13 -> ESCExtBrkAvail/1  "<ESCExtBrkAvail>"
  Bus Selector/12 -> ESCBrakStatus/1  "<ESCBrakStatus>"
  Bus Selector/11 -> EMSTqSrc/1  "<EMSTqSrc>"
  Bus Selector/10 -> EMSExtTqAvail/1  "<EMSExtTqAvail>"
  Bus Selector/9 -> DrivBrakSw/1  "<DrivBrakSw>"
  Bus Selector/8 -> DecContMan/1  "<DecContMan>"
  Bus Selector/7 -> CurVehDec_V/1  "<CurVehDec_V>"
  Bus Selector/6 -> CurVehDec/1  "<CurVehDec>"
  Bus Selector/4 -> CurEngTqReq/1  "<CurEngTqReq>"
  Bus Selector/2 -> CurBrakDecReq/1  "<CurBrakDecReq>"
  Bus Selector/1 -> BrakePrefillAvail/1  "<BrakePrefillAvail>"
  CAN1_Rx/1 -> [CAN1_Rx]
  [CAN1_Rx] -> Bus Selector/1

== system hal/dHAL_IN/HAL_IN_VCU/BO__1361_VCU2__8_VCU ==
  CAN1_Rx : Inport
  Bus Selector : BusSelector  OutputSignals=VCU2.VCU_AccelPedalPosn,VCU2.VCU_AccelPedalPosn_V,VCU2.CurDriverTqReq,VCU2.CurDriverTqReq_V,VCU2.VCU2_LifeCount,VCU2.VCU2_Checksum
  ChecksumCalculation : Subsystem  TreatAsAtomicUnit=on
  VCU_AccelPedalPosn : Outport
  VCU_AccelPedalPosn_V : Outport  Port=2
  CurDriverTqReq : Outport  Port=3
  CurDriverTqReq_V : Outport  Port=4
  VCU2_LifeCount : Outport  Port=5
  VCU2_Checksum : Outport  Port=6
  Message_Checksum : Outport  Port=7
  wires:
  Bus Selector/4 -> CurDriverTqReq_V/1  "<CurDriverTqReq_V>"
  Bus Selector/3 -> CurDriverTqReq/1  "<CurDriverTqReq>"
  Bus Selector/5 -> VCU2_LifeCount/1  "<VCU2_LifeCount>"
  Bus Selector/6 -> VCU2_Checksum/1  "<VCU2_Checksum>"
  Bus Selector/2 -> VCU_AccelPedalPosn_V/1  "<VCU_AccelPedalPosn_V>"
  Bus Selector/1 -> VCU_AccelPedalPosn/1  "<VCU_AccelPedalPosn>"
  ChecksumCalculation/1(Message_Checksum) -> Message_Checksum/1
  [CAN1_Rx] -> ChecksumCalculation/1(CAN1_Rx)
  [CAN1_Rx] -> Bus Selector/1
  CAN1_Rx/1 -> [CAN1_Rx]
